simulink model "Sistema_Seguimiento_Con_Planta_Tipo_0"  (R2016a)
settings: Solver=VariableStepAuto  StartTime=0.0  StopTime=30  RelTol=1e-3
values from neighbouring files (symbols this model uses):
  A = flip(fliplr(A))    [Ackerman_Ejemplo_Con_Tipo_0.m]
  B = flip(B)    [Ackerman_Ejemplo_Con_Tipo_0.m]
  C = fliplr(C)    [Ackerman_Ejemplo_Con_Tipo_0.m]
  Init_cond = [0 0 0]    [Ackerman_Con_cond_iniciales_SYM.m]    (also in Ackerman_Ejemplo_Con_Tipo_0.m)
undefined symbols (not defined in the file or in its folder): D
libraries: simulink x1
settings Model: Creator=adrie  LastModifiedBy=adrie
settings GRTTargetCC: GeneratePreprocessorConditionals=Use local settings

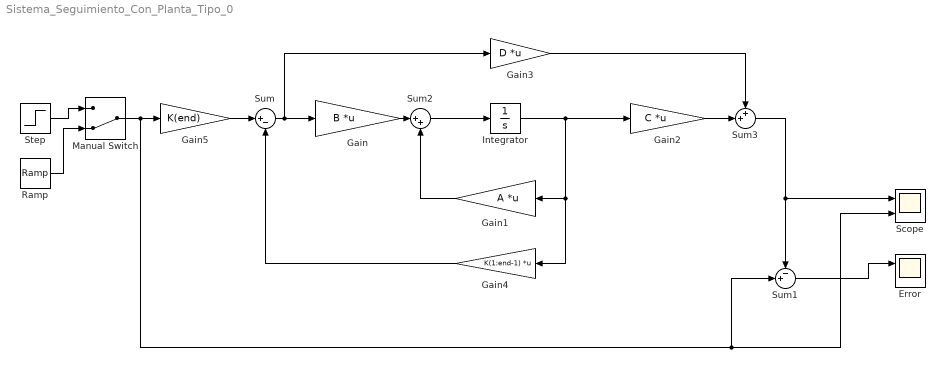
== system Sistema_Seguimiento_Con_Planta_Tipo_0 ==
  "Error " : Scope  NumInputPorts=2
  Gain : Gain  Gain=B  Multiplication=Matrix(K*u) (u vector)
  Gain1 : Gain  Gain=A  Multiplication=Matrix(K*u) (u vector)
  Gain2 : Gain  Gain=C  Multiplication=Matrix(K*u) (u vector)
  Gain3 : Gain  Gain=D  Multiplication=Matrix(K*u) (u vector)
  Gain4 : Gain  Gain=K(1:end-1)  Multiplication=Matrix(K*u) (u vector)
  Gain5 : Gain  Gain=K(end)
  Integrator : Integrator  InitialCondition=Init_cond
  Manual Switch : ManualSwitch  CurrentSetting=0
  Ramp : simulink/Sources/Ramp  slope=1  start=0  X0=0
  Scope : Scope  NumInputPorts=2
  Step : Step  Time=0  SampleTime=0
  Sum : Sum  Inputs=|+-
  Sum1 : Sum  Inputs=-+|
  Sum2 : Sum  Inputs=|++
  Sum3 : Sum  Inputs=++|
  wires:
  Gain/1 -> Sum2/1
  Sum2/1 -> Integrator/1
  Gain1/1 -> Sum2/2
  Integrator/1 -> Gain2/1, Gain4/1, Gain1/1
  Gain2/1 -> Sum3/2
  Gain3/1 -> Sum3/1
  Sum3/1 -> Sum1/1, Scope/1
  Sum/1 -> Gain3/1, Gain/1
  Gain4/1 -> Sum/2
  Step/1 -> Manual Switch/1
  Gain5/1 -> Sum/1
  Manual Switch/1 -> Sum1/2, Scope/2, Gain5/1
  Ramp/1 -> Manual Switch/2
  Sum1/1 -> "Error "/1
